simulink subsystem "MFTiresLongitudinal"  (R2023a)
settings: Solver=VariableStepAuto  StartTime=0.0  StopTime=10.0  RelTol=1e-3
libraries: autolibutils x2, autolibshared x2, autolibpowerinfoutils x2
(part 2 of 2)

== system MFTiresLongitudinal/Longitudinal Wheel - Front 2 ==
  Info : Inport
  Bus Selector : BusSelector  OutputSignals=PwrInfo.PwrTrnsfrd,PwrInfo.PwrNotTrnsfrd,PwrInfo.PwrStored
  Power Accounting Bus Creator : autolibpowerinfoutils/Power Accounting Bus Creator  AssctBlkSelPopup=Parent  RefBlkName='libraryname/blkname'  PwrTrnsfrdCheckBox=on  PwrNotTrnsfrdCheckBox=on  PwrStoredCheckBox=on  aMode=6
  Terminator3 : Terminator
  wires:
  Info/1 -> Bus Selector/1
  Bus Selector/1 -> Power Accounting Bus Creator/1  "<PwrTrnsfrd>"
  Bus Selector/2 -> Power Accounting Bus Creator/2  "<PwrNotTrnsfrd>"
  Bus Selector/3 -> Power Accounting Bus Creator/3  "<PwrStored>"
  Power Accounting Bus Creator/1 -> Terminator3/1

== system MFTiresLongitudinal/Longitudinal Wheel - Rear 2 ==
  Info : Inport
  Bus Selector : BusSelector  OutputSignals=PwrInfo.PwrTrnsfrd,PwrInfo.PwrNotTrnsfrd,PwrInfo.PwrStored
  Power Accounting Bus Creator : autolibpowerinfoutils/Power Accounting Bus Creator  AssctBlkSelPopup=Parent  RefBlkName='libraryname/blkname'  PwrTrnsfrdCheckBox=on  PwrNotTrnsfrdCheckBox=on  PwrStoredCheckBox=on  aMode=6
  Terminator3 : Terminator
  wires:
  Info/1 -> Bus Selector/1
  Bus Selector/1 -> Power Accounting Bus Creator/1  "<PwrTrnsfrd>"
  Bus Selector/2 -> Power Accounting Bus Creator/2  "<PwrNotTrnsfrd>"
  Bus Selector/3 -> Power Accounting Bus Creator/3  "<PwrStored>"
  Power Accounting Bus Creator/1 -> Terminator3/1

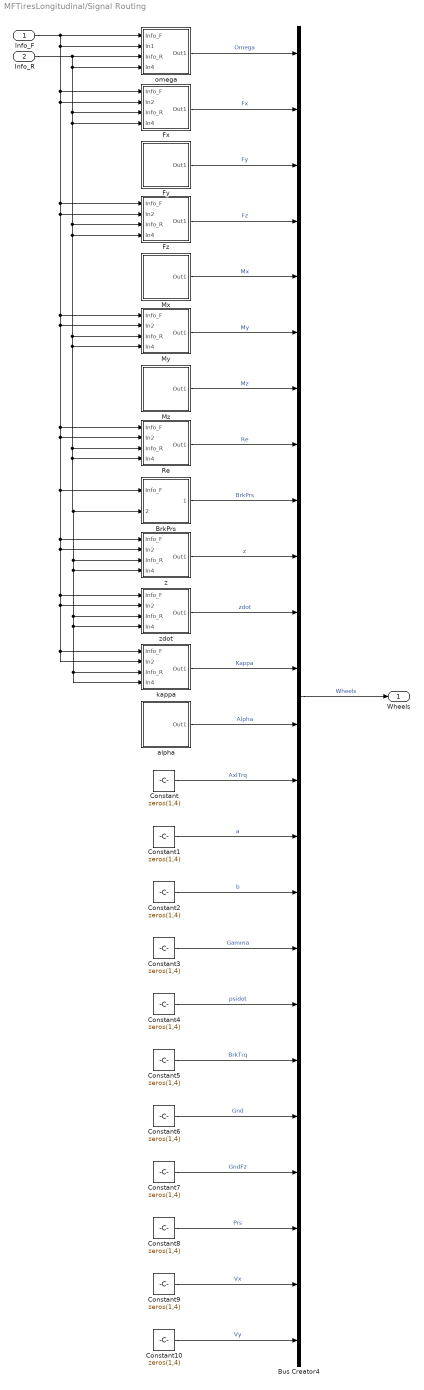
== system MFTiresLongitudinal/Signal Routing ==
  Info_F : Inport
  Info_R : Inport  Port=2
  BrkPrs : Subsystem
  Bus Creator4 : BusCreator  Inputs=24
  Constant{,1..10} (11 alike) : Constant  Value=zeros(1,4)  SampleTime=-1
  Fx : Subsystem
  Fy : Subsystem
  Fz : Subsystem
  Mx : Subsystem
  My : Subsystem
  Mz : Subsystem
  Re : Subsystem
  alpha : Subsystem
  kappa : Subsystem
  omega : Subsystem
  z : Subsystem
  zdot : Subsystem
  Wheels : Outport
  wires:
  Constant10/1 -> Bus Creator4/24  "Vy"
  Constant9/1 -> Bus Creator4/23  "Vx"
  Constant8/1 -> Bus Creator4/22  "Prs"
  Constant7/1 -> Bus Creator4/21  "GndFz"
  Constant6/1 -> Bus Creator4/20  "Gnd"
  Constant5/1 -> Bus Creator4/19  "BrkTrq"
  Constant4/1 -> Bus Creator4/18  "psidot"
  Constant3/1 -> Bus Creator4/17  "Gamma"
  Constant2/1 -> Bus Creator4/16  "b"
  Constant1/1 -> Bus Creator4/15  "a"
  Constant/1 -> Bus Creator4/14  "AxlTrq"
  BrkPrs/1(BrkPrs) -> Bus Creator4/9  "BrkPrs"
  Bus Creator4/1 -> Wheels/1  "Wheels"
  alpha/1(Out1) -> Bus Creator4/13  "Alpha"
  My/1(Out1) -> Bus Creator4/6  "My"
  Fy/1(Out1) -> Bus Creator4/3  "Fy"
  z/1(Out1) -> Bus Creator4/10  "z"
  omega/1(Out1) -> Bus Creator4/1  "Omega"
  Mz/1(Out1) -> Bus Creator4/7  "Mz"
  kappa/1(Out1) -> Bus Creator4/12  "Kappa"
  zdot/1(Out1) -> Bus Creator4/11  "zdot"
  Mx/1(Out1) -> Bus Creator4/5  "Mx"
  Fx/1(Out1) -> Bus Creator4/2  "Fx"
  Info_R/1 -> omega/3(Info_R), omega/4(In4), Fx/3(Info_R), Fx/4(In4), Fz/3(Info_R), Fz/4(In4), My/3(Info_R), My/4(In4), Re/3(Info_R), z/3(Info_R), z/4(In4), zdot/3(Info_R), zdot/4(In4), kappa/4(In4), kappa/3(Info_R), BrkPrs/2(Info_R), Re/4(In4)
  Info_F/1 -> omega/1(Info_F), Fz/1(Info_F), Fz/2(In2), My/1(Info_F), My/2(In2), Re/1(Info_F), Re/2(In2), z/1(Info_F), z/2(In2), zdot/2(In2), kappa/2(In2), kappa/1(Info_F), zdot/1(Info_F), BrkPrs/1(Info_F), Fx/2(In2), Fx/1(Info_F), omega/2(In1)
  Fz/1(Out1) -> Bus Creator4/4  "Fz"
  Re/1(Out1) -> Bus Creator4/8  "Re"

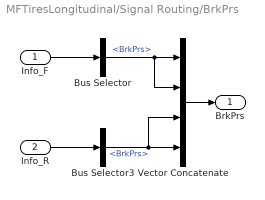
== system MFTiresLongitudinal/Signal Routing/BrkPrs ==
  Info_F : Inport
  Info_R : Inport  Port=2
  Bus Selector : BusSelector  OutputSignals=BrkPrs
  Bus Selector3 : BusSelector  OutputSignals=BrkPrs
  Vector Concatenate : Concatenate  NumInputs=4
  BrkPrs : Outport  PortDimensions=4  VectorParamsAs1DForOutWhenUnconnected=off
  wires:
  Bus Selector3/1 -> Vector Concatenate/4, Vector Concatenate/3  "<BrkPrs>"
  Vector Concatenate/1 -> BrkPrs/1
  Info_R/1 -> Bus Selector3/1
  Info_F/1 -> Bus Selector/1
  Bus Selector/1 -> Vector Concatenate/1, Vector Concatenate/2  "<BrkPrs>"

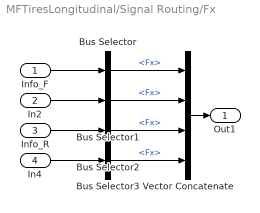
== system MFTiresLongitudinal/Signal Routing/Fx ==
  Info_F : Inport
  In2 : Inport  Port=2
  Info_R : Inport  Port=3
  In4 : Inport  Port=4
  Bus Selector{,1..3} (4 alike) : BusSelector  OutputSignals=Fx
  Vector Concatenate : Concatenate  NumInputs=4
  Out1 : Outport  PortDimensions=4  VectorParamsAs1DForOutWhenUnconnected=off
  wires:
  Bus Selector3/1 -> Vector Concatenate/4  "<Fx>"
  Bus Selector2/1 -> Vector Concatenate/3  "<Fx>"
  Bus Selector1/1 -> Vector Concatenate/2  "<Fx>"
  In4/1 -> Bus Selector3/1
  Info_R/1 -> Bus Selector2/1
  In2/1 -> Bus Selector1/1
  Bus Selector/1 -> Vector Concatenate/1  "<Fx>"
  Info_F/1 -> Bus Selector/1
  Vector Concatenate/1 -> Out1/1

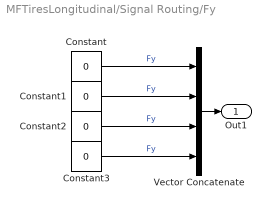
== system MFTiresLongitudinal/Signal Routing/Fy ==
  Constant{,1..3} (4 alike) : Constant  Value=0  SampleTime=-1
  Vector Concatenate : Concatenate  NumInputs=4
  Out1 : Outport  PortDimensions=4  VectorParamsAs1DForOutWhenUnconnected=off
  wires:
  Constant3/1 -> Vector Concatenate/4  "Fy"
  Constant2/1 -> Vector Concatenate/3  "Fy"
  Constant1/1 -> Vector Concatenate/2  "Fy"
  Vector Concatenate/1 -> Out1/1
  Constant/1 -> Vector Concatenate/1  "Fy"

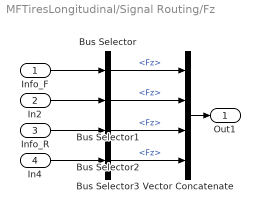
== system MFTiresLongitudinal/Signal Routing/Fz ==
  Info_F : Inport
  In2 : Inport  Port=2
  Info_R : Inport  Port=3
  In4 : Inport  Port=4
  Bus Selector{,1..3} (4 alike) : BusSelector  OutputSignals=Fz
  Vector Concatenate : Concatenate  NumInputs=4
  Out1 : Outport  PortDimensions=4  VectorParamsAs1DForOutWhenUnconnected=off
  wires:
  Vector Concatenate/1 -> Out1/1
  Info_F/1 -> Bus Selector/1
  Bus Selector/1 -> Vector Concatenate/1  "<Fz>"
  In2/1 -> Bus Selector1/1
  Info_R/1 -> Bus Selector2/1
  In4/1 -> Bus Selector3/1
  Bus Selector1/1 -> Vector Concatenate/2  "<Fz>"
  Bus Selector2/1 -> Vector Concatenate/3  "<Fz>"
  Bus Selector3/1 -> Vector Concatenate/4  "<Fz>"

== system MFTiresLongitudinal/Signal Routing/Mx ==
  Constant{,1..3} (4 alike) : Constant  Value=0  SampleTime=-1
  Vector Concatenate : Concatenate  NumInputs=4
  Out1 : Outport  PortDimensions=4  VectorParamsAs1DForOutWhenUnconnected=off
  wires:
  Constant2/1 -> Vector Concatenate/3  "Mx"
  Constant3/1 -> Vector Concatenate/4  "Mx"
  Constant/1 -> Vector Concatenate/1  "Mx"
  Constant1/1 -> Vector Concatenate/2  "Mx"
  Vector Concatenate/1 -> Out1/1

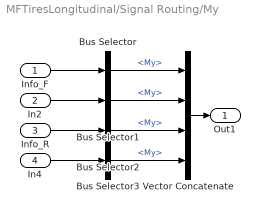
== system MFTiresLongitudinal/Signal Routing/My ==
  Info_F : Inport
  In2 : Inport  Port=2
  Info_R : Inport  Port=3
  In4 : Inport  Port=4
  Bus Selector{,1..3} (4 alike) : BusSelector  OutputSignals=My
  Vector Concatenate : Concatenate  NumInputs=4
  Out1 : Outport  PortDimensions=4  VectorParamsAs1DForOutWhenUnconnected=off
  wires:
  Bus Selector3/1 -> Vector Concatenate/4  "<My>"
  Bus Selector2/1 -> Vector Concatenate/3  "<My>"
  Bus Selector1/1 -> Vector Concatenate/2  "<My>"
  In4/1 -> Bus Selector3/1
  Info_R/1 -> Bus Selector2/1
  In2/1 -> Bus Selector1/1
  Bus Selector/1 -> Vector Concatenate/1  "<My>"
  Info_F/1 -> Bus Selector/1
  Vector Concatenate/1 -> Out1/1

== system MFTiresLongitudinal/Signal Routing/Mz ==
  Constant{,1..3} (4 alike) : Constant  Value=0  SampleTime=-1
  Vector Concatenate : Concatenate  NumInputs=4
  Out1 : Outport  PortDimensions=4  VectorParamsAs1DForOutWhenUnconnected=off
  wires:
  Constant2/1 -> Vector Concatenate/3  "Mz"
  Constant3/1 -> Vector Concatenate/4  "Mz"
  Constant/1 -> Vector Concatenate/1  "Mz"
  Constant1/1 -> Vector Concatenate/2  "Mz"
  Vector Concatenate/1 -> Out1/1

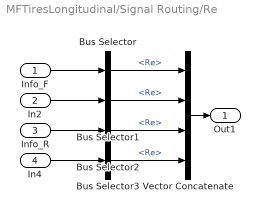
== system MFTiresLongitudinal/Signal Routing/Re ==
  Info_F : Inport
  In2 : Inport  Port=2
  Info_R : Inport  Port=3
  In4 : Inport  Port=4
  Bus Selector{,1..3} (4 alike) : BusSelector  OutputSignals=Re
  Vector Concatenate : Concatenate  NumInputs=4
  Out1 : Outport  PortDimensions=4  VectorParamsAs1DForOutWhenUnconnected=off
  wires:
  Vector Concatenate/1 -> Out1/1
  Info_F/1 -> Bus Selector/1
  Bus Selector/1 -> Vector Concatenate/1  "<Re>"
  In2/1 -> Bus Selector1/1
  Info_R/1 -> Bus Selector2/1
  In4/1 -> Bus Selector3/1
  Bus Selector1/1 -> Vector Concatenate/2  "<Re>"
  Bus Selector2/1 -> Vector Concatenate/3  "<Re>"
  Bus Selector3/1 -> Vector Concatenate/4  "<Re>"

== system MFTiresLongitudinal/Signal Routing/alpha ==
  Constant{,1..3} (4 alike) : Constant  Value=0  SampleTime=-1
  Vector Concatenate : Concatenate  NumInputs=4
  Out1 : Outport  PortDimensions=4  VectorParamsAs1DForOutWhenUnconnected=off
  wires:
  Constant2/1 -> Vector Concatenate/3  "Alpha"
  Constant3/1 -> Vector Concatenate/4  "Alpha"
  Constant/1 -> Vector Concatenate/1  "Alpha"
  Constant1/1 -> Vector Concatenate/2  "Alpha"
  Vector Concatenate/1 -> Out1/1

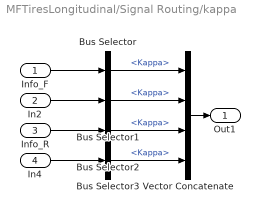
== system MFTiresLongitudinal/Signal Routing/kappa ==
  Info_F : Inport
  In2 : Inport  Port=2
  Info_R : Inport  Port=3
  In4 : Inport  Port=4
  Bus Selector{,1..3} (4 alike) : BusSelector  OutputSignals=Kappa
  Vector Concatenate : Concatenate  NumInputs=4
  Out1 : Outport  PortDimensions=4  VectorParamsAs1DForOutWhenUnconnected=off
  wires:
  Bus Selector3/1 -> Vector Concatenate/4  "<Kappa>"
  Bus Selector2/1 -> Vector Concatenate/3  "<Kappa>"
  Bus Selector1/1 -> Vector Concatenate/2  "<Kappa>"
  In4/1 -> Bus Selector3/1
  Info_R/1 -> Bus Selector2/1
  In2/1 -> Bus Selector1/1
  Bus Selector/1 -> Vector Concatenate/1  "<Kappa>"
  Info_F/1 -> Bus Selector/1
  Vector Concatenate/1 -> Out1/1

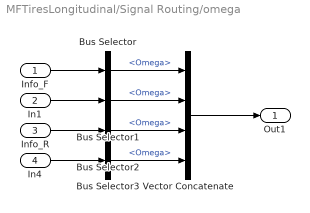
== system MFTiresLongitudinal/Signal Routing/omega ==
  Info_F : Inport
  In1 : Inport  Port=2
  Info_R : Inport  Port=3
  In4 : Inport  Port=4
  Bus Selector{,1..3} (4 alike) : BusSelector  OutputSignals=Omega
  Vector Concatenate : Concatenate  NumInputs=4
  Out1 : Outport  PortDimensions=4  VectorParamsAs1DForOutWhenUnconnected=off
  wires:
  Info_F/1 -> Bus Selector/1
  Bus Selector/1 -> Vector Concatenate/1  "<Omega>"
  In1/1 -> Bus Selector1/1
  Info_R/1 -> Bus Selector2/1
  In4/1 -> Bus Selector3/1
  Bus Selector1/1 -> Vector Concatenate/2  "<Omega>"
  Bus Selector2/1 -> Vector Concatenate/3  "<Omega>"
  Bus Selector3/1 -> Vector Concatenate/4  "<Omega>"
  Vector Concatenate/1 -> Out1/1

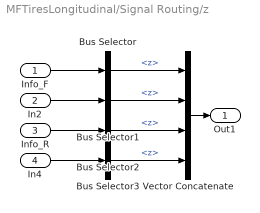
== system MFTiresLongitudinal/Signal Routing/z ==
  Info_F : Inport
  In2 : Inport  Port=2
  Info_R : Inport  Port=3
  In4 : Inport  Port=4
  Bus Selector{,1..3} (4 alike) : BusSelector  OutputSignals=z
  Vector Concatenate : Concatenate  NumInputs=4
  Out1 : Outport  PortDimensions=4  VectorParamsAs1DForOutWhenUnconnected=off
  wires:
  Bus Selector3/1 -> Vector Concatenate/4  "<z>"
  Bus Selector2/1 -> Vector Concatenate/3  "<z>"
  Bus Selector1/1 -> Vector Concatenate/2  "<z>"
  In4/1 -> Bus Selector3/1
  Info_R/1 -> Bus Selector2/1
  In2/1 -> Bus Selector1/1
  Bus Selector/1 -> Vector Concatenate/1  "<z>"
  Info_F/1 -> Bus Selector/1
  Vector Concatenate/1 -> Out1/1

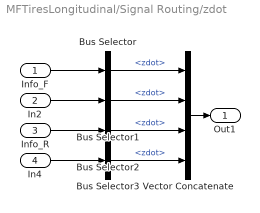
== system MFTiresLongitudinal/Signal Routing/zdot ==
  Info_F : Inport
  In2 : Inport  Port=2
  Info_R : Inport  Port=3
  In4 : Inport  Port=4
  Bus Selector{,1..3} (4 alike) : BusSelector  OutputSignals=zdot
  Vector Concatenate : Concatenate  NumInputs=4
  Out1 : Outport  PortDimensions=4  VectorParamsAs1DForOutWhenUnconnected=off
  wires:
  Vector Concatenate/1 -> Out1/1
  Info_F/1 -> Bus Selector/1
  Bus Selector/1 -> Vector Concatenate/1  "<zdot>"
  In2/1 -> Bus Selector1/1
  Info_R/1 -> Bus Selector2/1
  In4/1 -> Bus Selector3/1
  Bus Selector1/1 -> Vector Concatenate/2  "<zdot>"
  Bus Selector2/1 -> Vector Concatenate/3  "<zdot>"
  Bus Selector3/1 -> Vector Concatenate/4  "<zdot>"
